simulink model "Automatic_Laser_Follower_Project"  (R2023b)
settings: Solver=ode45  StartTime=0.0  StopTime=100.0  RelTol=1e-3  EnableMultiTasking=on
undefined symbols (not defined in the file): fspecial, gray, none, Rec, SDTV, videoinput
libraries: visiontextngfix x11, visionconversions x4, visionanalysis x4, visionstatistics x3, simulink x3, imaqlib x1
settings Model: SimulationMode=accelerator  Creator=Chris  LastModifiedBy=fanyi
settings SolverCC: AlgebraicLoopSolver=TrustRegion
settings DataIOCC: LimitDataPoints=on  SaveFormat=Array  SignalLoggingSaveFormat=ModelDataLogs  ReturnWorkspaceOutputs=off
settings OptimizationCC: ExpressionDepthLimit=2147483647  LifeSpan=inf
settings DebuggingCC: UnderspecifiedInitializationDetection=Classic  MergeDetectMultiDrivingBlocksExec=none  SolverPrmCheckMsg=warning  FcnCallInpInsideContextMsg=warning  UnconnectedInputMsg=warning  UnconnectedOutputMsg=warning  UnconnectedLineMsg=warning  StateNameClashWarn=warning  SFUnexpectedBacktrackingDiag=warning  SFNoUnconditionalDefaultTransitionDiag=warning  SFExecutionAtInitializationDiag=none  ArithmeticOperatorsInVariantConditions=warning
settings HardwareCC: ProdBitPerPointer=32  ProdBitPerSizeT=32  ProdBitPerPtrDiffT=32  ProdLargestAtomicFloat=None  ProdIntDivRoundTo=Undefined  ProdEndianess=Unspecified  ProdWordSize=32  ProdHWDeviceType=32-bit Generic
settings ModelReferenceCC: EnableRefExpFcnMdlSchedulingChecks=on  PropagateSignalLabelsOutOfModel=off
settings SFSimCC: SimUseLocalCustomCode=off  CustomCodeUndefinedFunction=UseInterfaceOnly
settings RTWCC: RTWUseLocalCustomCode=off  DLArmComputeVersion=19.05
settings CodeAppCC: StateflowObjectComments=on
settings GRTTargetCC: TargetLangStandard=C89/C90 (ANSI)  CombineOutputUpdateFcns=off  GRTInterface=on
settings ConfigComp: CovMetricSettings=dw  CovSaveCumulativeToWorkspaceVar=on  CovSaveSingleToWorkspaceVar=on  CovExternalEMLEnable=off

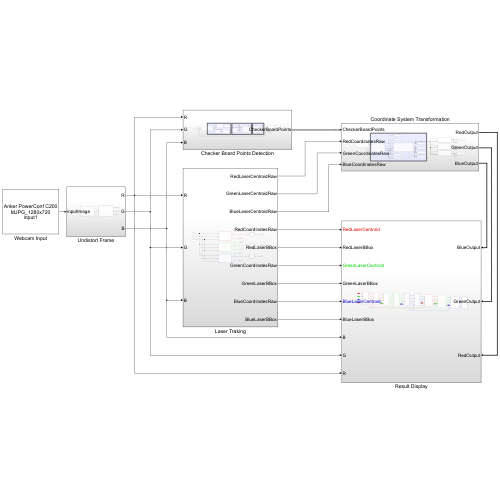
[thumbnail: Simulink's stored preview of the top-level diagram]
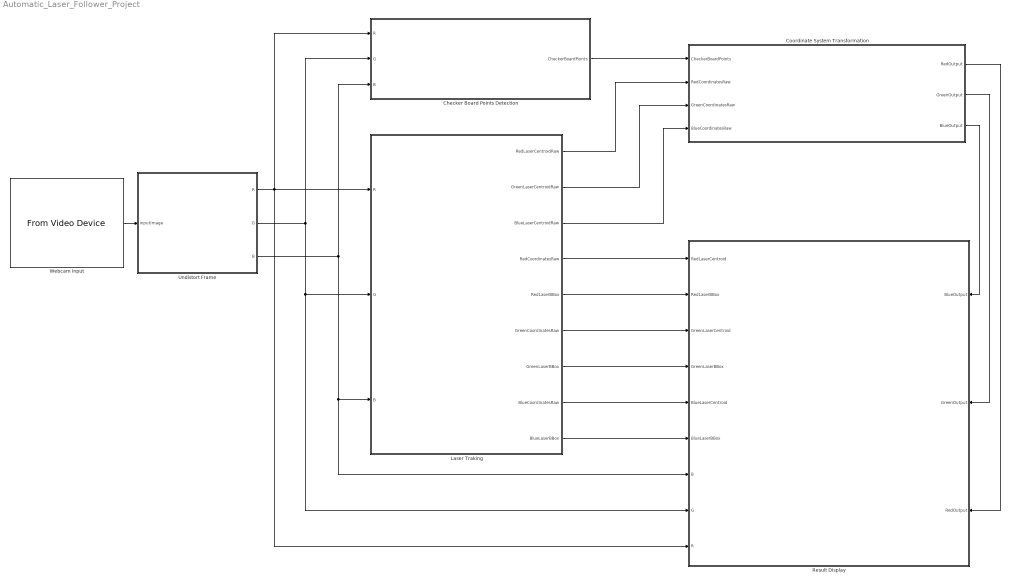
== system Automatic_Laser_Follower_Project ==
  Checker Board Points Detection : Subsystem
  Coordinate System Transformation : Subsystem
  Laser Traking : Subsystem
  Result Display : Subsystem
      settings: PortSchema="{\"entries\":[{\"content\":{\"sides\":[{\"content\":{\"connectorIds\":[\"In1\",\"In2\",\"In3\",\"In4\",\"In5\",\"In6\",\"In7\",\"In8\",\"In9\"]},\"type\":\"ConnectorPlacement.EquallySpacedRectSide\",\"uuid\":\"b1906bfe-0566-47b0-9e68-516326f7bec6\"},{\"content\":{\"connectorIds\":[\"In10\",\"In11\",\"In12\"],\"side\":\"RIGHT\"},\"type\":\"ConnectorPlacement.EquallySpacedRectSide\",\"uuid\":\"6258ed97-87fe-4cc0-87ce-9e8e3abb5e56\"},{\"content\":{\"side\":\"TOP\"},\"type\":\"ConnectorPlacement.EquallySpacedRectSide\",\"uuid\":\"7eb9bd65-632c-4cad-bc7f-e4ae4268f70b\"}]},\"type\":\"ConnectorPlacement.EquallySpacedConnector\",\"uuid\":\"5d2784b2-c65f-4f4f-828d-caa1666124b0\"}],\"packageUris\":[\"http://schema.mathworks.com/mf0/Connector/R2020b\"],\"version\":\"1.0\"}"
  Undistort Frame : Subsystem
  Webcam Input : imaqlib/From Video Device  DeviceMenu=winvideo 1 (Anker PowerConf C200)  Device=winvideo 1 (Anker PowerConf C200)  ObjConstructor=videoinput('winvideo', 1)  VideoFormatMenu=MJPG_1280x720  VideoFormat=MJPG_1280x720  VideoSource=input1  ROIPosition=[0 0 720 1280]  EnableHWTrigger=off  TriggerConfiguration=none/none  SampleTime=1/30  OutputPortsMode=One multidimensional signal  DataType=single  CanDoHWTrigger=no  ReturnedColorSpace=rgb  BlockHandle=1881.0001  ROIWidth=1280  ROIHeight=720  ROIColumn=0  ROIRow=0  EngXMLPath=C:\Program Files\MATLAB\R2023b\toolbox\imaq\imaq\private  DevXMLPath=C:\ProgramData\MATLAB\SupportPackages\R2023b\toolbox\imaq\supportpackages\genericvideo\adaptor\win64  EngLibPath=C:\Program Files\MATLAB\R2023b\toolbox\imaq\imaqblks\imaqmex\win64  ColorSpace=rgb  BayerSensorAlignment=grbg  ImaqMode=off
  wires:
  Checker Board Points Detection/1(CheckerBoardPoints) -> Coordinate System Transformation/1(CheckerBoardPoints)
  Coordinate System Transformation/1(RedOutput) -> Result Display/12(RedOutput)
  Coordinate System Transformation/3(BlueOutput) -> Result Display/10(BlueOutput)
  Coordinate System Transformation/2(GreenOutput) -> Result Display/11(GreenOutput)
  Laser Traking/4(RedCoordinatesRaw) -> Result Display/1(RedLaserCentroid)
  Laser Traking/5(RedLaserBBox) -> Result Display/2(RedLaserBBox)
  Laser Traking/6(GreenCoordinatesRaw) -> Result Display/3(GreenLaserCentroid)
  Laser Traking/7(GreenLaserBBox) -> Result Display/4(GreenLaserBBox)
  Laser Traking/8(BlueCoordinatesRaw) -> Result Display/5(BlueLaserCentroid)
  Laser Traking/9(BlueLaserBBox) -> Result Display/6(BlueLaserBBox)
  Laser Traking/1(RedLaserCentroidRaw) -> Coordinate System Transformation/2(RedCoordinatesRaw)
  Laser Traking/2(GreenLaserCentroidRaw) -> Coordinate System Transformation/3(GreenCoordinatesRaw)
  Laser Traking/3(BlueLaserCentroidRaw) -> Coordinate System Transformation/4(BlueCoordinatesRaw)
  Webcam Input/1 -> Undistort Frame/1(inputImage)
  Undistort Frame/2(G) -> Checker Board Points Detection/2(G), Result Display/8(G), Laser Traking/2(G)
  Undistort Frame/1(R) -> Checker Board Points Detection/1(R), Result Display/9(R), Laser Traking/1(R)
  Undistort Frame/3(B) -> Checker Board Points Detection/3(B), Result Display/7(B), Laser Traking/3(B)

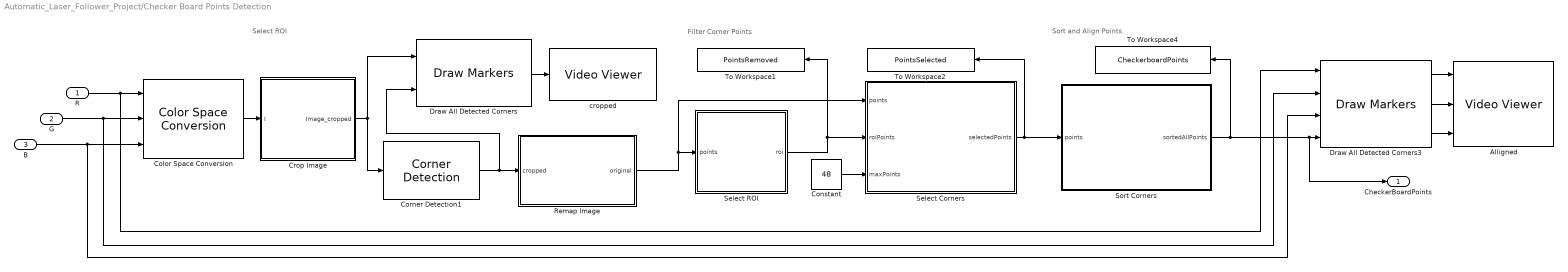
== system Automatic_Laser_Follower_Project/Checker Board Points Detection ==
  note: Sort and Align Points
  note: Select ROI
  note: Filter Corner Points
  R : Inport
  G : Inport  Port=2
  B : Inport  Port=3
  Alligned : VideoViewer  imagePorts=separate color signals  colormapValue=gray(256)  FigPos=[629.666666666667 1316.66666666667 1589.33333333333 1111.33333333333]
  Color Space Conversion : visionconversions/Color Space  Conversion  conversion=Obsolete  conversionActive=R'G'B' to intensity  wp_str=D65  rec=Rec. 601 (SDTV)  sys=1125/60/2:1  imagePorts=Separate color signals
  Constant : Constant  Value=48
  Corner Detection1 : visionanalysis/Corner Detection  method=Harris corner detection (Harris & Stephens)  factor=0.1  filter=fspecial('gaussian', [1 5], 1.5)  thrInten=0.1  thrAngle=157.5  output=Obsolete9b  outputInUse=Corner location  maxNum=80  thrMetric=0.0004  neighborSize=[21 21]  isOutVarDim=on  roundingMode=Floor  overflowMode=off  firstCoeffMode=Specify word length  firstCoeffWordLength=16  firstCoeffFracLength=16  prodOutputMode=Binary point scaling  prodOutputWordLength=32  prodOutputFracLength=0  accumMode=Binary point scaling  accumWordLength=32  accumFracLength=0  memoryMode=Binary point scaling  memoryWordLength=32  memoryFracLength=0
  Crop Image : MATLAB Function  TreatAsAtomicUnit=on
  Draw All Detected Corners : visiontextngfix/Draw Markers  shape=Circle  size=2  fill=on  fillClrSource=Specify via dialog  display=User-specified value  intensity=200  color=[250 0 0]  opacity=0.6  viewport=Entire image  antialiasing=off  inType=Obsolete  imagePorts=One multidimensional signal  roundingMode=Floor  overflowMode=off  memoryMode=Specify word length  memoryWordLength=16  memoryFracLength=15  prodOutputMode=Binary point scaling  prodOutputWordLength=32  prodOutputFracLength=14
  Draw All Detected Corners3 : visiontextngfix/Draw Markers  shape=Circle  size=2  fill=on  fillClrSource=Specify via dialog  display=User-specified value  intensity=200  color=[250 0 0]  opacity=0.6  viewport=Entire image  antialiasing=off  inType=Obsolete  imagePorts=Separate color signals  roundingMode=Floor  overflowMode=off  memoryMode=Specify word length  memoryWordLength=16  memoryFracLength=15  prodOutputMode=Binary point scaling  prodOutputWordLength=32  prodOutputFracLength=14
  Remap Image : MATLAB Function  TreatAsAtomicUnit=on
  Select Corners : MATLAB Function  TreatAsAtomicUnit=on
  Select ROI : MATLAB Function  TreatAsAtomicUnit=on
  Sort Corners : MATLAB Function  TreatAsAtomicUnit=on
  To Workspace1 : ToWorkspace  VariableName=PointsRemoved  SaveFormat=Structure With Time  SampleTime=-1
      settings: Save2DSignal=2-D array (concatenate along first dimension)
  To Workspace2 : ToWorkspace  VariableName=PointsSelected  SaveFormat=Structure With Time  SampleTime=-1
      settings: Save2DSignal=2-D array (concatenate along first dimension)
  To Workspace4 : ToWorkspace  VariableName=CheckerboardPoints  SaveFormat=Structure With Time  SampleTime=-1
      settings: Save2DSignal=2-D array (concatenate along first dimension)
  cropped : VideoViewer  colormapValue=gray(256)  FigPos=[1282.33333333333 1388.66666666667 1277.33333333333 1286]
  CheckerBoardPoints : Outport
  wires:
  G/1 -> Color Space Conversion/2, Draw All Detected Corners3/2
  B/1 -> Color Space Conversion/3, Draw All Detected Corners3/3
  R/1 -> Color Space Conversion/1, Draw All Detected Corners3/1
  Select ROI/1(roi) -> To Workspace1/1, Select Corners/2(roiPoints)
  Constant/1 -> Select Corners/3(maxPoints)
  Draw All Detected Corners3/2 -> Alligned/2
  Draw All Detected Corners3/3 -> Alligned/3
  Draw All Detected Corners3/1 -> Alligned/1
  Select Corners/1(selectedPoints) -> To Workspace2/1, Sort Corners/1(points)
  Draw All Detected Corners/1 -> cropped/1
  Color Space Conversion/1 -> Crop Image/1(I)
  Remap Image/1(original) -> Select Corners/1(points), Select ROI/1(points)
  Crop Image/1(Image_cropped) -> Corner Detection1/1, Draw All Detected Corners/1
  Corner Detection1/1 -> Remap Image/1(cropped), Draw All Detected Corners/2
  Sort Corners/1(sortedAllPoints) -> To Workspace4/1, Draw All Detected Corners3/4, CheckerBoardPoints/1

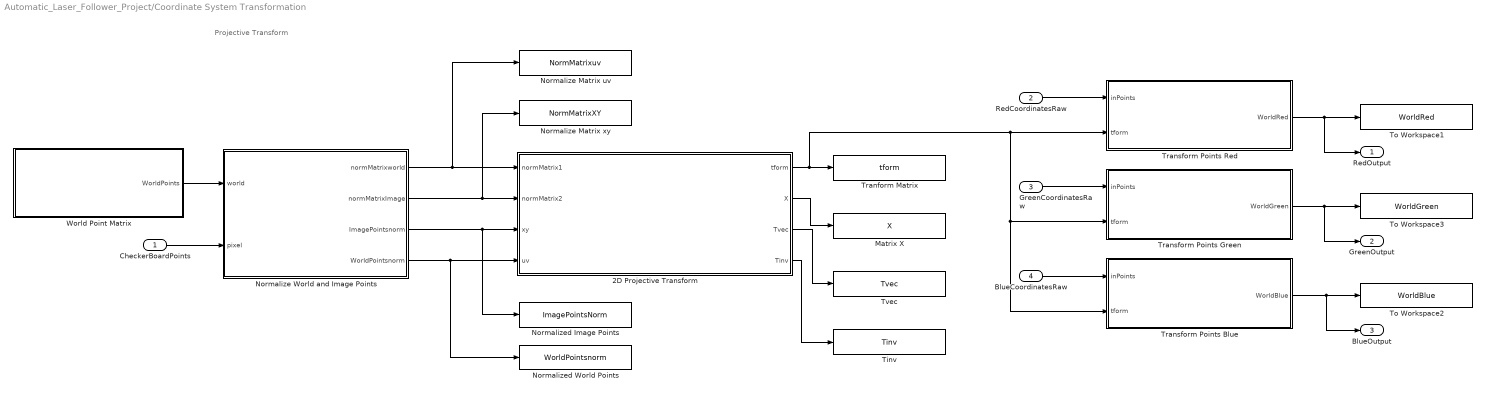
== system Automatic_Laser_Follower_Project/Coordinate System Transformation ==
  note: Projective Transform
  CheckerBoardPoints : Inport
  RedCoordinatesRaw : Inport  Port=2
  GreenCoordinatesRaw : Inport  Port=3
  BlueCoordinatesRaw : Inport  Port=4
  2D Projective Transform : MATLAB Function  TreatAsAtomicUnit=on
  Matrix X : ToWorkspace  VariableName=X  SaveFormat=Structure With Time  SampleTime=-1
      settings: Save2DSignal=2-D array (concatenate along first dimension)
  Normalize Matrix uv : ToWorkspace  VariableName=NormMatrixuv  SaveFormat=Structure With Time  SampleTime=-1
      settings: Save2DSignal=2-D array (concatenate along first dimension)
  Normalize Matrix xy : ToWorkspace  VariableName=NormMatrixXY  SaveFormat=Structure With Time  SampleTime=-1
      settings: Save2DSignal=2-D array (concatenate along first dimension)
  Normalize World and Image Points : MATLAB Function  TreatAsAtomicUnit=on
  Normalized Image Points : ToWorkspace  VariableName=ImagePointsNorm  SaveFormat=Structure With Time  SampleTime=-1
      settings: Save2DSignal=2-D array (concatenate along first dimension)
  Normalized World Points : ToWorkspace  VariableName=WorldPointsnorm  SaveFormat=Structure With Time  SampleTime=-1
      settings: Save2DSignal=2-D array (concatenate along first dimension)
  Tinv : ToWorkspace  VariableName=Tinv  SaveFormat=Structure With Time  SampleTime=-1
      settings: Save2DSignal=2-D array (concatenate along first dimension)
  To Workspace1 : ToWorkspace  VariableName=WorldRed  SaveFormat=Structure With Time  SampleTime=-1
      settings: Save2DSignal=2-D array (concatenate along first dimension)
  To Workspace2 : ToWorkspace  VariableName=WorldBlue  SaveFormat=Structure With Time  SampleTime=-1
      settings: Save2DSignal=2-D array (concatenate along first dimension)
  To Workspace3 : ToWorkspace  VariableName=WorldGreen  SaveFormat=Structure With Time  SampleTime=-1
      settings: Save2DSignal=2-D array (concatenate along first dimension)
  Tranform Matrix : ToWorkspace  VariableName=tform  SaveFormat=Structure With Time  SampleTime=-1
      settings: Save2DSignal=2-D array (concatenate along first dimension)
  Transform Points Blue : MATLAB Function  TreatAsAtomicUnit=on
  Transform Points Green : MATLAB Function  TreatAsAtomicUnit=on
  Transform Points Red : MATLAB Function  TreatAsAtomicUnit=on
  Tvec : ToWorkspace  VariableName=Tvec  SaveFormat=Structure With Time  SampleTime=-1
      settings: Save2DSignal=2-D array (concatenate along first dimension)
  World Point Matrix : MATLAB Function  TreatAsAtomicUnit=on
  RedOutput : Outport
  GreenOutput : Outport  Port=2
  BlueOutput : Outport  Port=3
  wires:
  Transform Points Red/1(WorldRed) -> RedOutput/1, To Workspace1/1
  Transform Points Green/1(WorldGreen) -> GreenOutput/1, To Workspace3/1
  Transform Points Blue/1(WorldBlue) -> To Workspace2/1, BlueOutput/1
  RedCoordinatesRaw/1 -> Transform Points Red/1(inPoints)
  GreenCoordinatesRaw/1 -> Transform Points Green/1(inPoints)
  BlueCoordinatesRaw/1 -> Transform Points Blue/1(inPoints)
  2D Projective Transform/1(tform) -> Tranform Matrix/1, Transform Points Blue/2(tform), Transform Points Green/2(tform), Transform Points Red/2(tform)
  CheckerBoardPoints/1 -> Normalize World and Image Points/2(pixel)
  Normalize World and Image Points/4(WorldPointsnorm) -> 2D Projective Transform/4(uv), Normalized World Points/1
  Normalize World and Image Points/2(normMatrixImage) -> Normalize Matrix xy/1, 2D Projective Transform/2(normMatrix2)
  Normalize World and Image Points/1(normMatrixworld) -> Normalize Matrix uv/1, 2D Projective Transform/1(normMatrix1)
  World Point Matrix/1(WorldPoints) -> Normalize World and Image Points/1(world)
  Normalize World and Image Points/3(ImagePointsnorm) -> Normalized Image Points/1, 2D Projective Transform/3(xy)
  2D Projective Transform/2(X) -> Matrix X/1
  2D Projective Transform/3(Tvec) -> Tvec/1
  2D Projective Transform/4(Tinv) -> Tinv/1

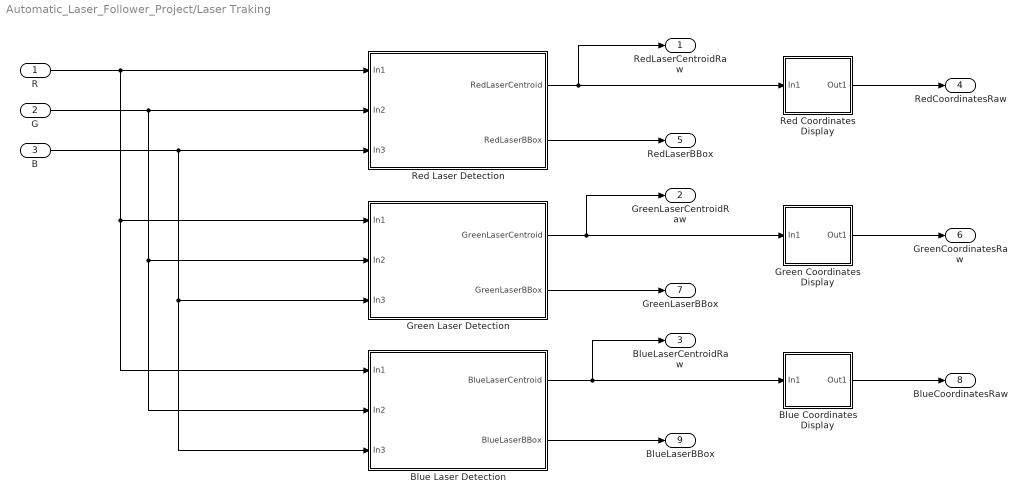
== system Automatic_Laser_Follower_Project/Laser Traking ==
  R : Inport
  G : Inport  Port=2
  B : Inport  Port=3
  Blue Coordinates Display : Subsystem
  Blue Laser Detection : Subsystem
  Green Coordinates Display : Subsystem
  Green Laser Detection : Subsystem
  Red Coordinates Display : Subsystem
  Red Laser Detection : Subsystem  VariantControl=Choice
  RedLaserCentroidRaw : Outport
  GreenLaserCentroidRaw : Outport  Port=2
  BlueLaserCentroidRaw : Outport  Port=3
  RedCoordinatesRaw : Outport  Port=4
  RedLaserBBox : Outport  Port=5
  GreenCoordinatesRaw : Outport  Port=6
  GreenLaserBBox : Outport  Port=7
  BlueCoordinatesRaw : Outport  Port=8
  BlueLaserBBox : Outport  Port=9
  wires:
  Blue Laser Detection/2(BlueLaserBBox) -> BlueLaserBBox/1
  Green Laser Detection/1(GreenLaserCentroid) -> Green Coordinates Display/1(In1), GreenLaserCentroidRaw/1
  Red Laser Detection/1(RedLaserCentroid) -> Red Coordinates Display/1(In1), RedLaserCentroidRaw/1
  Blue Laser Detection/1(BlueLaserCentroid) -> BlueLaserCentroidRaw/1, Blue Coordinates Display/1(In1)
  Red Laser Detection/2(RedLaserBBox) -> RedLaserBBox/1
  Red Coordinates Display/1(Out1) -> RedCoordinatesRaw/1
  Green Coordinates Display/1(Out1) -> GreenCoordinatesRaw/1
  Blue Coordinates Display/1(Out1) -> BlueCoordinatesRaw/1
  G/1 -> Green Laser Detection/2(In2), Blue Laser Detection/2(In2), Red Laser Detection/2(In2)
  Green Laser Detection/2(GreenLaserBBox) -> GreenLaserBBox/1
  R/1 -> Blue Laser Detection/1(In1), Green Laser Detection/1(In1), Red Laser Detection/1(In1)
  B/1 -> Blue Laser Detection/3(In3), Green Laser Detection/3(In3), Red Laser Detection/3(In3)

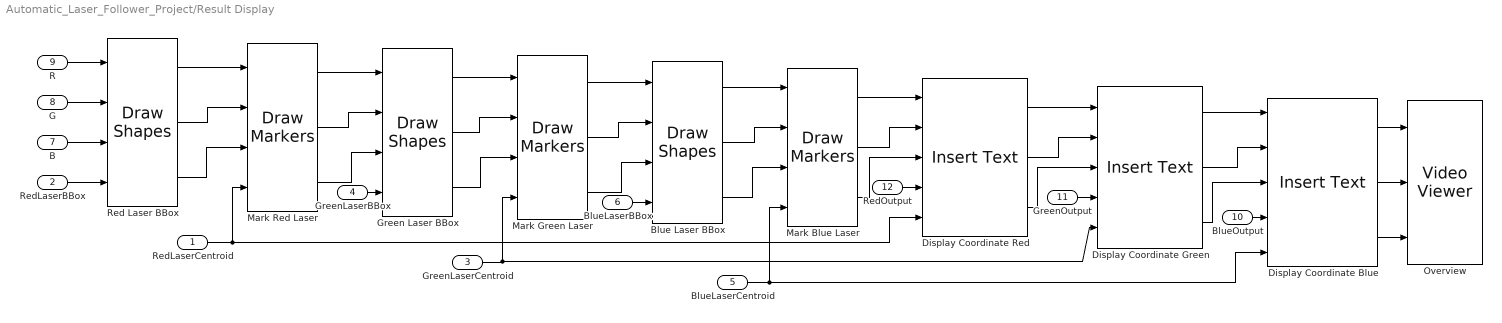
== system Automatic_Laser_Follower_Project/Result Display ==
  RedLaserCentroid : Inport
  RedLaserBBox : Inport  Port=2
  GreenLaserCentroid : Inport  Port=3
  GreenLaserBBox : Inport  Port=4
  BlueLaserCentroid : Inport  Port=5
  BlueLaserBBox : Inport  Port=6
  B : Inport  Port=7
  G : Inport  Port=8
  R : Inport  Port=9
  BlueOutput : Inport  Port=10
  GreenOutput : Inport  Port=11
  RedOutput : Inport  Port=12
  Blue Laser BBox : visiontextngfix/Draw Shapes  shape=Rectangles  fill=off  lineWidth=3  fillClrSource=Specify via dialog  display=User-specified value  intensity=200  color=[0 0 255]  opacity=0.6  viewport=Entire image  antialiasing=off  inType=Obsolete  imagePorts=Separate color signals  roundingMode=Floor  overflowMode=off  memoryMode=Specify word length  memoryWordLength=16  prodOutputMode=Binary point scaling  prodOutputWordLength=32  prodOutputFracLength=14  memoryFracLength=15
  Display Coordinate Blue : visiontextngfix/Insert Text  inputType=Obsolete  theText='blue: %.3f mm, %.3f mm'  getTextLocFrom=Input port  textLoc=[1 1]  getTextColorFrom=Specify via dialog  textColor=[0 0 255]  getTextIntensityFrom=Specify via dialog  textIntensity=0  getTextOpacityFrom=Specify via dialog  textOpacity=1.0  dummyVar2=0  dummyVar3=0  dummyVar4=0  imagePorts=Separate color signals  isInputTransposed=off  fontFace=LucidaSansRegular  dummyVar1=0  blockFontSize=18  antiAliased=on
  Display Coordinate Green : visiontextngfix/Insert Text  inputType=Obsolete  theText='Green: %.3f mm, %.3f mm'  getTextLocFrom=Input port  textLoc=[1 1]  getTextColorFrom=Specify via dialog  textColor=[0 255 0]  getTextIntensityFrom=Specify via dialog  textIntensity=0  getTextOpacityFrom=Specify via dialog  textOpacity=1.0  dummyVar2=0  dummyVar3=0  dummyVar4=0  imagePorts=Separate color signals  isInputTransposed=off  fontFace=LucidaSansRegular  dummyVar1=0  blockFontSize=18  antiAliased=on
  Display Coordinate Red : visiontextngfix/Insert Text  inputType=Obsolete  theText='Red: %.3f mm, %.3f mm'  getTextLocFrom=Input port  textLoc=[1 1]  getTextColorFrom=Specify via dialog  textColor=[255 0 0]  getTextIntensityFrom=Specify via dialog  textIntensity=0  getTextOpacityFrom=Specify via dialog  textOpacity=1.0  dummyVar2=0  dummyVar3=0  dummyVar4=0  imagePorts=Separate color signals  isInputTransposed=off  fontFace=LucidaSansRegular  dummyVar1=0  blockFontSize=18  antiAliased=on
  Green Laser BBox : visiontextngfix/Draw Shapes  shape=Rectangles  fill=off  lineWidth=3  fillClrSource=Specify via dialog  display=User-specified value  intensity=200  color=[0 255 0]  opacity=0.6  viewport=Entire image  antialiasing=off  inType=Obsolete  imagePorts=Separate color signals  roundingMode=Floor  overflowMode=off  memoryMode=Specify word length  memoryWordLength=16  prodOutputMode=Binary point scaling  prodOutputWordLength=32  prodOutputFracLength=14  memoryFracLength=15
  Mark Blue Laser : visiontextngfix/Draw Markers  shape=X-mark  size=5  fill=on  fillClrSource=Specify via dialog  display=User-specified value  intensity=200  color=[0 0 255]  opacity=0.6  viewport=Entire image  antialiasing=off  inType=Obsolete  imagePorts=Separate color signals  roundingMode=Floor  overflowMode=off  memoryMode=Specify word length  memoryWordLength=16  memoryFracLength=15  prodOutputMode=Binary point scaling  prodOutputWordLength=32  prodOutputFracLength=14
  Mark Green Laser : visiontextngfix/Draw Markers  shape=X-mark  size=5  fill=on  fillClrSource=Specify via dialog  display=User-specified value  intensity=200  color=[0 255 0]  opacity=0.6  viewport=Entire image  antialiasing=off  inType=Obsolete  imagePorts=Separate color signals  roundingMode=Floor  overflowMode=off  memoryMode=Specify word length  memoryWordLength=16  memoryFracLength=15  prodOutputMode=Binary point scaling  prodOutputWordLength=32  prodOutputFracLength=14
  Mark Red Laser : visiontextngfix/Draw Markers  shape=X-mark  size=5  fill=on  fillClrSource=Specify via dialog  display=User-specified value  intensity=200  color=[255 0 0]  opacity=0.6  viewport=Entire image  antialiasing=off  inType=Obsolete  imagePorts=Separate color signals  roundingMode=Floor  overflowMode=off  memoryMode=Specify word length  memoryWordLength=16  memoryFracLength=15  prodOutputMode=Binary point scaling  prodOutputWordLength=32  prodOutputFracLength=14
  Overview : VideoViewer  imagePorts=separate color signals  colormapValue=gray(256)  FigPos=[1 1390 2560 1294.66666666667]
  Red Laser BBox : visiontextngfix/Draw Shapes  shape=Rectangles  fill=off  lineWidth=3  fillClrSource=Specify via dialog  display=User-specified value  intensity=200  color=[255 0 0]  opacity=0.6  viewport=Entire image  antialiasing=off  inType=Obsolete  imagePorts=Separate color signals  roundingMode=Floor  overflowMode=off  memoryMode=Specify word length  memoryWordLength=16  prodOutputMode=Binary point scaling  prodOutputWordLength=32  prodOutputFracLength=14  memoryFracLength=15
  wires:
  RedLaserBBox/1 -> Red Laser BBox/4
  Mark Green Laser/1 -> Blue Laser BBox/1
  Green Laser BBox/3 -> Mark Green Laser/3
  Mark Green Laser/2 -> Blue Laser BBox/2
  Mark Green Laser/3 -> Blue Laser BBox/3
  Display Coordinate Green/3 -> Display Coordinate Blue/3
  Mark Blue Laser/1 -> Display Coordinate Red/1
  Green Laser BBox/1 -> Mark Green Laser/1
  Display Coordinate Green/2 -> Display Coordinate Blue/2
  Display Coordinate Red/1 -> Display Coordinate Green/1
  Blue Laser BBox/1 -> Mark Blue Laser/1
  Display Coordinate Green/1 -> Display Coordinate Blue/1
  Blue Laser BBox/3 -> Mark Blue Laser/3
  Red Laser BBox/3 -> Mark Red Laser/3
  Red Laser BBox/2 -> Mark Red Laser/2
  Mark Red Laser/3 -> Green Laser BBox/3
  Mark Blue Laser/2 -> Display Coordinate Red/2
  Mark Red Laser/2 -> Green Laser BBox/2
  Green Laser BBox/2 -> Mark Green Laser/2
  Red Laser BBox/1 -> Mark Red Laser/1
  Display Coordinate Red/3 -> Display Coordinate Green/3
  RedLaserCentroid/1 -> Mark Red Laser/4, Display Coordinate Red/5
  Blue Laser BBox/2 -> Mark Blue Laser/2
  Display Coordinate Red/2 -> Display Coordinate Green/2
  R/1 -> Red Laser BBox/1
  Mark Blue Laser/3 -> Display Coordinate Red/3
  BlueLaserBBox/1 -> Blue Laser BBox/4
  B/1 -> Red Laser BBox/3
  GreenLaserBBox/1 -> Green Laser BBox/4
  Mark Red Laser/1 -> Green Laser BBox/1
  GreenLaserCentroid/1 -> Display Coordinate Green/5, Mark Green Laser/4
  BlueLaserCentroid/1 -> Mark Blue Laser/4, Display Coordinate Blue/5
  G/1 -> Red Laser BBox/2
  Display Coordinate Blue/1 -> Overview/1
  Display Coordinate Blue/2 -> Overview/2
  Display Coordinate Blue/3 -> Overview/3
  RedOutput/1 -> Display Coordinate Red/4
  BlueOutput/1 -> Display Coordinate Blue/4
  GreenOutput/1 -> Display Coordinate Green/4

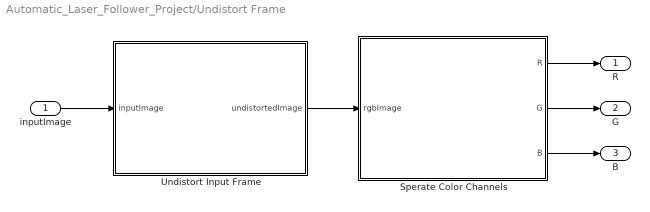
== system Automatic_Laser_Follower_Project/Undistort Frame ==
  inputImage : Inport
  Sperate Color Channels : MATLAB Function  TreatAsAtomicUnit=on
  Undistort Input Frame : MATLAB Function  TreatAsAtomicUnit=on
  R : Outport
  G : Outport  Port=2
  B : Outport  Port=3
  wires:
  Sperate Color Channels/2(G) -> G/1
  Sperate Color Channels/3(B) -> B/1
  Sperate Color Channels/1(R) -> R/1
  inputImage/1 -> Undistort Input Frame/1(inputImage)
  Undistort Input Frame/1(undistortedImage) -> Sperate Color Channels/1(rgbImage)

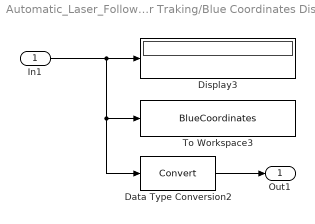
== system Automatic_Laser_Follower_Project/Laser Traking/Blue Coordinates Display ==
  In1 : Inport
  Data Type Conversion2 : DataTypeConversion  ConvertRealWorld=Stored Integer (SI)  SaturateOnIntegerOverflow=off  RndMeth=Floor
  Display3 : Display
  To Workspace3 : ToWorkspace  VariableName=BlueCoordinates  SampleTime=-1
      settings: Save2DSignal=2-D array (concatenate along first dimension)
  Out1 : Outport
  wires:
  In1/1 -> Data Type Conversion2/1, To Workspace3/1, Display3/1
  Data Type Conversion2/1 -> Out1/1

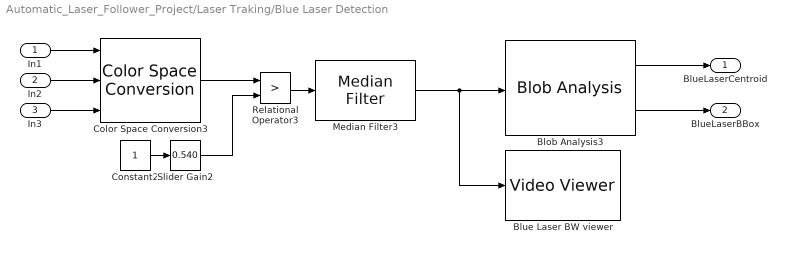
== system Automatic_Laser_Follower_Project/Laser Traking/Blue Laser Detection ==
  In1 : Inport
  In2 : Inport  Port=2
  In3 : Inport  Port=3
  Blob Analysis3 : visionstatistics/Blob Analysis  Tag=vipblks_row_conv  area=off  centroid=on  bBox=on  majorAxis=off  minorAxis=off  angle=off  eccentricity=off  equivDiameterSq=off  extent=off  perimeter=off  outDT=double  conn=8  isLabel=off  maxBlobs=1  warnIfNumBlobsExceeded=on  isCount=off  useMinArea=on  minArea=40  useMaxArea=on  maxArea=intmax('uint32')  excludeBorderBlob=off  isOutVarDim=off  isFill=on  fillValues=-1  roundingMode=Floor  overflowMode=off  prodOutputMode=Binary point scaling  prodOutputWordLength=32  prodOutputFracLength=16  accumMode=Binary point scaling  accumWordLength=32  accumFracLength=0  outputMode=Binary point scaling  outputWordLength=32  outputFracLength=16  firstCoeffMode=Binary point scaling  firstCoeffWordLength=16  firstCoeffFracLength=14  secondCoeffMode=Binary point scaling  secondCoeffWordLength=32  secondCoeffFracLength=16
  Blue Laser BW viewer : VideoViewer  colormapValue=gray(256)  FigPos=[933 1177.33333333333 1538 856.666666666667]
  Color Space Conversion3 : visionconversions/Color Space  Conversion  conversion=Obsolete  conversionActive=R'G'B' to Y'CbCr  wp_str=D65  rec=Rec. 601 (SDTV)  sys=1125/60/2:1  imagePorts=Separate color signals
  Constant2 : Constant
  Median Filter3 : visionanalysis/Median Filter  nghbood=ones(1, 1)  outSize=Valid  padType=Constant  padSrc=Specify via dialog  padVal=0  roundingMode=Floor  overflowMode=off
  Relational Operator3 : RelationalOperator  Operator=>  OutDataTypeStr=boolean  RndMeth=Simplest  InputSameDT=off
  Slider Gain2 : simulink/Math Operations/Slider Gain  gain=0.540  low=0  high=1
  BlueLaserCentroid : Outport
  BlueLaserBBox : Outport  Port=2
  wires:
  Slider Gain2/1 -> Relational Operator3/2
  Median Filter3/1 -> Blob Analysis3/1, Blue Laser BW viewer/1
  In2/1 -> Color Space Conversion3/2
  Constant2/1 -> Slider Gain2/1
  Relational Operator3/1 -> Median Filter3/1
  Color Space Conversion3/2 -> Relational Operator3/1
  Blob Analysis3/1 -> BlueLaserCentroid/1
  In1/1 -> Color Space Conversion3/1
  Blob Analysis3/2 -> BlueLaserBBox/1
  In3/1 -> Color Space Conversion3/3

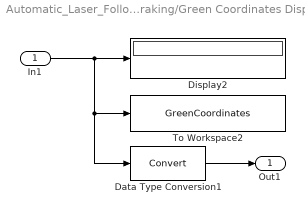
== system Automatic_Laser_Follower_Project/Laser Traking/Green Coordinates Display ==
  In1 : Inport
  Data Type Conversion1 : DataTypeConversion  ConvertRealWorld=Stored Integer (SI)  SaturateOnIntegerOverflow=off  RndMeth=Floor
  Display2 : Display
  To Workspace2 : ToWorkspace  VariableName=GreenCoordinates  SampleTime=-1
      settings: Save2DSignal=2-D array (concatenate along first dimension)
  Out1 : Outport
  wires:
  Data Type Conversion1/1 -> Out1/1
  In1/1 -> Data Type Conversion1/1, To Workspace2/1, Display2/1

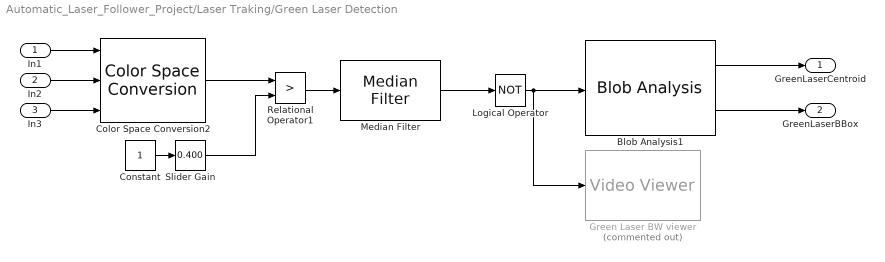
== system Automatic_Laser_Follower_Project/Laser Traking/Green Laser Detection ==
  In1 : Inport
  In2 : Inport  Port=2
  In3 : Inport  Port=3
  Blob Analysis1 : visionstatistics/Blob Analysis  Tag=vipblks_row_conv  area=off  centroid=on  bBox=on  majorAxis=off  minorAxis=off  angle=off  eccentricity=off  equivDiameterSq=off  extent=off  perimeter=off  outDT=double  conn=8  isLabel=off  maxBlobs=1  warnIfNumBlobsExceeded=on  isCount=off  useMinArea=on  minArea=0  useMaxArea=on  maxArea=intmax('uint32')  excludeBorderBlob=off  isOutVarDim=off  isFill=on  fillValues=-1  roundingMode=Floor  overflowMode=off  prodOutputMode=Binary point scaling  prodOutputWordLength=32  prodOutputFracLength=16  accumMode=Binary point scaling  accumWordLength=32  accumFracLength=0  outputMode=Binary point scaling  outputWordLength=32  outputFracLength=16  firstCoeffMode=Binary point scaling  firstCoeffWordLength=16  firstCoeffFracLength=14  secondCoeffMode=Binary point scaling  secondCoeffWordLength=32  secondCoeffFracLength=16
  Color Space Conversion2 : visionconversions/Color Space  Conversion  conversion=Obsolete  conversionActive=R'G'B' to Y'CbCr  wp_str=D65  rec=Rec. 601 (SDTV)  sys=1125/60/2:1  imagePorts=Separate color signals
  Constant : Constant
  Green Laser BW viewer : VideoViewer  Commented=on  colormapValue=gray(256)  FigPos=[991.666666666667 959.333333333333 1476 664]
  Logical Operator : Logic  Operator=NOT  AllPortsSameDT=off  OutDataTypeStr=boolean
  Median Filter : visionanalysis/Median Filter  nghbood=ones(1, 1)  outSize=Valid  padType=Constant  padSrc=Specify via dialog  padVal=0  roundingMode=Floor  overflowMode=off
  Relational Operator1 : RelationalOperator  Operator=>  OutDataTypeStr=boolean  RndMeth=Simplest  InputSameDT=off
  Slider Gain : simulink/Math Operations/Slider Gain  gain=0.400  low=0  high=1
  GreenLaserCentroid : Outport
  GreenLaserBBox : Outport  Port=2
  wires:
  Blob Analysis1/2 -> GreenLaserBBox/1
  Relational Operator1/1 -> Median Filter/1
  Slider Gain/1 -> Relational Operator1/2
  Median Filter/1 -> Logical Operator/1
  Color Space Conversion2/2 -> Relational Operator1/1
  In3/1 -> Color Space Conversion2/3
  Constant/1 -> Slider Gain/1
  In2/1 -> Color Space Conversion2/2
  In1/1 -> Color Space Conversion2/1
  Blob Analysis1/1 -> GreenLaserCentroid/1
  Logical Operator/1 -> Green Laser BW viewer/1, Blob Analysis1/1

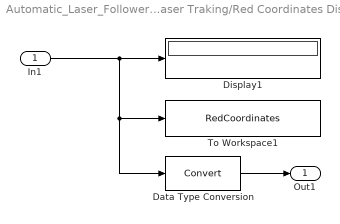
== system Automatic_Laser_Follower_Project/Laser Traking/Red Coordinates Display ==
  In1 : Inport
  Data Type Conversion : DataTypeConversion  ConvertRealWorld=Stored Integer (SI)  SaturateOnIntegerOverflow=off  RndMeth=Floor
  Display1 : Display
  To Workspace1 : ToWorkspace  VariableName=RedCoordinates  SampleTime=-1
      settings: Save2DSignal=2-D array (concatenate along first dimension)
  Out1 : Outport
  wires:
  In1/1 -> Data Type Conversion/1, To Workspace1/1, Display1/1
  Data Type Conversion/1 -> Out1/1

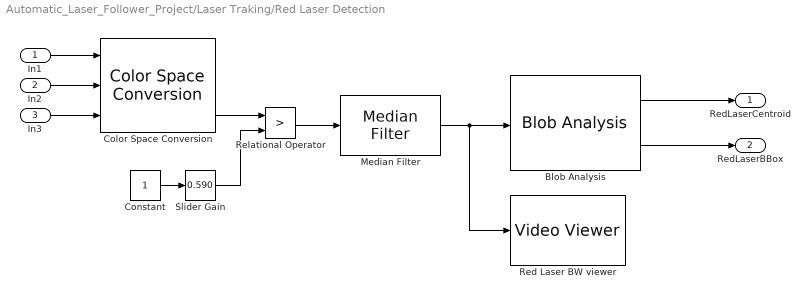
== system Automatic_Laser_Follower_Project/Laser Traking/Red Laser Detection ==
  In1 : Inport
  In2 : Inport  Port=2
  In3 : Inport  Port=3
  Blob Analysis : visionstatistics/Blob Analysis  Tag=vipblks_row_conv  area=off  centroid=on  bBox=on  majorAxis=off  minorAxis=off  angle=off  eccentricity=off  equivDiameterSq=off  extent=off  perimeter=off  outDT=double  conn=8  isLabel=off  maxBlobs=1  warnIfNumBlobsExceeded=on  isCount=off  useMinArea=on  minArea=0  useMaxArea=on  maxArea=intmax('uint32')  excludeBorderBlob=off  isOutVarDim=off  isFill=on  fillValues=-1  roundingMode=Floor  overflowMode=off  prodOutputMode=Binary point scaling  prodOutputWordLength=32  prodOutputFracLength=16  accumMode=Binary point scaling  accumWordLength=32  accumFracLength=0  outputMode=Binary point scaling  outputWordLength=32  outputFracLength=16  firstCoeffMode=Binary point scaling  firstCoeffWordLength=16  firstCoeffFracLength=14  secondCoeffMode=Binary point scaling  secondCoeffWordLength=32  secondCoeffFracLength=16
  Color Space Conversion : visionconversions/Color Space  Conversion  conversion=Obsolete  conversionActive=R'G'B' to Y'CbCr  wp_str=D65  rec=Rec. 601 (SDTV)  sys=1125/60/2:1  imagePorts=Separate color signals
  Constant : Constant
  Median Filter : visionanalysis/Median Filter  nghbood=ones(1, 1)  outSize=Valid  padType=Constant  padSrc=Specify via dialog  padVal=0  roundingMode=Floor  overflowMode=off
  Red Laser BW viewer : VideoViewer  colormapValue=gray(256)  FigPos=[9 1382 2544 1278.66666666667]
  Relational Operator : RelationalOperator  Operator=>  OutDataTypeStr=boolean  RndMeth=Simplest  InputSameDT=off
  Slider Gain : simulink/Math Operations/Slider Gain  gain=0.590  low=0  high=1
  RedLaserCentroid : Outport
  RedLaserBBox : Outport  Port=2
  wires:
  In2/1 -> Color Space Conversion/2
  In3/1 -> Color Space Conversion/3
  Median Filter/1 -> Blob Analysis/1, Red Laser BW viewer/1
  Relational Operator/1 -> Median Filter/1
  Constant/1 -> Slider Gain/1
  Slider Gain/1 -> Relational Operator/2
  Color Space Conversion/3 -> Relational Operator/1
  Blob Analysis/2 -> RedLaserBBox/1
  In1/1 -> Color Space Conversion/1
  Blob Analysis/1 -> RedLaserCentroid/1

== matlab function Automatic_Laser_Follower_Project/Coordinate System Transformation/Transform Points Red ==
  data: inPoints input; WorldRed output size=[1;2]; tform input
function WorldRed = TransformPointsInverseRed(inPoints, tform)

invtform = inv(tform);

homogPoints = [inPoints, ones(size(inPoints, 1), 1)];

transformedPoints = homogPoints * invtform'; 

% Normalize back to Cartesian coordinates
WorldRed = transformedPoints(:, 1:2) ./ transformedPoints(:, 3);


end

== matlab function Automatic_Laser_Follower_Project/Coordinate System Transformation/Transform Points Green ==
  data: inPoints input; WorldGreen output size=[1;2]; tform input
function WorldGreen = TransformPointsInverseGreen(inPoints, tform)

invtform = inv(tform);

homogPoints = [inPoints, ones(size(inPoints, 1), 1)];

transformedPoints = homogPoints * invtform'; 

% Normalize back to Cartesian coordinates
WorldGreen = transformedPoints(:, 1:2) ./ transformedPoints(:, 3);


end

== matlab function Automatic_Laser_Follower_Project/Checker Board Points Detection/Select Corners ==
  data: points input; roiPoints input size=[80;2]; selectedPoints output size=[80 2]; maxPoints input
function selectedPoints = selectCorners(points, roiPoints, maxPoints)
    %#codegen
    
    % Ensures the inputs are in the correct format
    assert(size(points, 2) == size(roiPoints, 2));
    
    % Using setdiff to find the points not in the ROI 
    selectedPoints = setdiff(points, roiPoints, 'rows', 'stable');
    
    % Makes sure the points selected does not overflow  
    if size(selectedPoints, 1) > maxPoints
        selectedPoints = selectedPoints(1:maxPoints, :);
    end
end

== matlab function Automatic_Laser_Follower_Project/Checker Board Points Detection/Select ROI ==
  data: points input size=[80;2]; roi output uint32 size=[80;2]
function roi = selectROI(points)
    %#codegen
    assert(size(points, 2) == 2, 'Input points must have exactly two columns'); % Assert input size
    
    points = double(points);
    
    % Calculates the convex hull of the points detected
    K = convhull(points(:,1), points(:,2));
    
    % Initialize a array for points touching or close to the convex hull
    isTouchingHull = false(size(points, 1), 1);
    
    % Define a threshold distance for points to be excluded in the ROI 
    threshold = 10; 

    % Loop over each segment of the convex hull
    for i = 1:numel(K)-1
        P1 = points(K(i), :);
        P2 = points(K(i+1), :);
        edgeVector = P2 - P1;

        for j = 1:size(points, 1)
            if ~isTouchingHull(j) % Only check points not already touching the hull
                pointVector = points(j, :) - P1;
                crossVec = norm(cross([pointVector 0], [edgeVector 0]));
                edgeLength = norm(edgeVector);
                distanceToEdge = crossVec / edgeLength;

                if distanceToEdge < threshold
                    isTouchingHull(j) = true;
                end
            end
        end
    end

    % Include points that are part of the hull or touching the hull
    isTouchingHull(K) = true;

    % Extract the points based on the logical index to be excluded in ROI 
    roiPoints = points(isTouchingHull, :);

    roi = uint32(roiPoints);
    
    assert(size(roi, 2) == 2);
end

== matlab function Automatic_Laser_Follower_Project/Checker Board Points Detection/Sort Corners ==
  data: points input; sortedAllPoints output size=[48;2]
function sortedAllPoints = sortCheckerboardPoints(points)
    points = double(points);

    % Remove rows with NaN values to clean the input data
    points = points(~any(isnan(points), 2), :);

    numRows = 6; 
    numCols = 8; 

    % Initialize the sorted points array
    sortedAllPoints = NaN(numRows * numCols, 2); 
    
    % Use kmeans to cluster points based on x-coordinate with PlusPlus initialization
    opts = statset('UseParallel', true, 'MaxIter', 1000);
    [idx, C] = kmeans(points(:,1), numCols, 'Options', opts, 'Distance', 'sqEuclidean', 'Replicates', 5, 'Start', 'plus');

    % Sort the centroids of clusters to ensure the order of clusters is from left to right
    [~, centroidOrder] = sort(C);
    
    % Initialize an index to keep track of where to insert points into sortedAllPoints
    insertIndex = 1;
    
    % Sort points within each cluster based on y-coordinate
    for i = 1:numCols
        % Find the points in the current cluster
        clusterPoints = points(idx == centroidOrder(i), :);
        
        % Sort the points in this cluster by their y-coordinate
        [~, order] = sort(clusterPoints(:,2), 'ascend');
        sortedClusterPoints = clusterPoints(order, :);
            
    % Dynamically handle missing or extra points in a cluster
    numPointsInCluster = size(sortedClusterPoints, 1);
    if numPointsInCluster >= numRows
        % If there are enough points, take the top numRows points
        sortedClusterPoints = sortedClusterPoints(1:numRows, :);
    else
        % If there are missing points, append NaN rows to make up the difference
        rowsToAdd = numRows - numPointsInCluster;
        if rowsToAdd > 0
            nanRows = NaN(rowsToAdd, 2);
            sortedClusterPoints = [sortedClusterPoints; nanRows];
        end
    end
        
        % Insert sorted points into the sortedAllPoints array
        sortedAllPoints(insertIndex:insertIndex + numRows - 1, :) = sortedClusterPoints;
        insertIndex = insertIndex + numRows;
    end
end

== matlab function Automatic_Laser_Follower_Project/Undistort Frame/Sperate Color Channels ==
  data: rgbImage input; R output; G output; B output
function [R, G, B] = separateColorChannels(rgbImage)
    % Check if the input image is indeed an RGB image
    if size(rgbImage, 3) ~= 3
        error('Input must be an RGB image.');
    end

    % Separate the color channels
    R = rgbImage(:, :, 1); 
    G = rgbImage(:, :, 2);  
    B = rgbImage(:, :, 3);  
end

== matlab function Automatic_Laser_Follower_Project/Checker Board Points Detection/Crop Image ==
  data: I input; Image_cropped output
function Image_cropped = cropImage(I)
    % cropping region
    rowStart = 300;
    rowEnd = 600;
    colStart = 300;
    colEnd = 600;

    Image_cropped = I(rowStart:rowEnd, colStart:colEnd);
end

== matlab function Automatic_Laser_Follower_Project/Checker Board Points Detection/Remap Image ==
  data: cropped input; original output size=[80;2]
function original = mapPointsToOriginal(cropped)
    rowOffset = 300 - 1;
    colOffset = 300 - 1;
    
    original = zeros(size(cropped));
    
    % Map each cropped point back to its original position
    for i = 1:size(cropped, 1)
        original(i, 1) = cropped(i, 1) + colOffset;
        original(i, 2) = cropped(i, 2) + rowOffset;
    end
end

== matlab function Automatic_Laser_Follower_Project/Undistort Frame/Undistort Input Frame ==
  data: inputImage input; undistortedImage output
function undistortedImage = undistortImage(inputImage)
    % Store the intrinsic matrix K
    intrinsicMatrix = [1025.30186847282, 0, 659.328530484529;
                       0, 1028.22633873043, 350.911761479516;
                       0, 0, 1];
    
    % Store the radial distortion coefficients
    k1 = 0.146451856840480;
    k2 = -0.129982636042747;
    
    % Initialize the undistorted image
    undistortedImage = zeros(size(inputImage), 'like', inputImage);
    
    % Get the number of rows and columns in the image
    [rows, cols, ~] = size(inputImage);
    
    for u = 1:cols
        for v = 1:rows
            % Convert pixel coordinates to normalized image coordinates
            x = (u - intrinsicMatrix(1,3)) / intrinsicMatrix(1,1);
            y = (v - intrinsicMatrix(2,3)) / intrinsicMatrix(2,2);
            
            % Compute the radius squared
            rSquared = x^2 + y^2;
            
            % Compute the undistortion factor
            undistortFactor = 1 + k1 * rSquared + k2 * rSquared^2;
            
            % Compute the undistorted coordinates
            xUndistorted = x * undistortFactor;
            yUndistorted = y * undistortFactor;
            
            % Convert back to pixel coordinates
            uUndistorted = round(xUndistorted * intrinsicMatrix(1,1) + intrinsicMatrix(1,3));
            vUndistorted = round(yUndistorted * intrinsicMatrix(2,2) + intrinsicMatrix(2,3));
            
            % Ensure the coordinates are within the image bounds
            if (uUndistorted > 0 && uUndistorted <= cols && vUndistorted > 0 && vUndistorted <= rows)
                undistortedImage(v, u, :) = inputImage(vUndistorted, uUndistorted, :);
            end
        end
    end
end

== matlab function Automatic_Laser_Follower_Project/Coordinate System Transformation/Transform Points Blue ==
  data: inPoints input; WorldBlue output size=[1;2]; tform input
function WorldBlue = TransformPointsInverseBlue(inPoints, tform)

invtform = inv(tform);

homogPoints = [inPoints, ones(size(inPoints, 1), 1)];

transformedPoints = homogPoints * invtform'; 

% Normalize back to Cartesian coordinates
WorldBlue = transformedPoints(:, 1:2) ./ transformedPoints(:, 3);


end

== matlab function Automatic_Laser_Follower_Project/Coordinate System Transformation/World Point Matrix ==
  data: WorldPoints output
function WorldPoints = StoreWorldPoints
% Update the square size to 29
squareSize = 29;

WorldPoints = [ ...
    0, 0;
    0, -squareSize;
    0, -2*squareSize;
    0, -3*squareSize;
    0, -4*squareSize;
    0, -5*squareSize;
    squareSize, 0;
    squareSize, -squareSize;
    squareSize, -2*squareSize;
    squareSize, -3*squareSize;
    squareSize, -4*squareSize;
    squareSize, -5*squareSize;
    2*squareSize, 0;
    2*squareSize, -squareSize;
    2*squareSize, -2*squareSize;
    2*squareSize, -3*squareSize;
    2*squareSize, -4*squareSize;
    2*squareSize, -5*squareSize;
    3*squareSize, 0;
    3*squareSize, -squareSize;
    3*squareSize, -2*squareSize;
    3*squareSize, -3*squareSize;
    3*squareSize, -4*squareSize;
    3*squareSize, -5*squareSize;
    4*squareSize, 0;
    4*squareSize, -squareSize;
    4*squareSize, -2*squareSize;
    4*squareSize, -3*squareSize;
    4*squareSize, -4*squareSize;
    4*squareSize, -5*squareSize;
    5*squareSize, 0;
    5*squareSize, -squareSize;
    5*squareSize, -2*squareSize;
    5*squareSize, -3*squareSize;
    5*squareSize, -4*squareSize;
    5*squareSize, -5*squareSize;
    6*squareSize, 0;
    6*squareSize, -squareSize;
    6*squareSize, -2*squareSize;
    6*squareSize, -3*squareSize;
    6*squareSize, -4*squareSize;
    6*squareSize, -5*squareSize;
    7*squareSize, 0;
    7*squareSize, -squareSize;
    7*squareSize, -2*squareSize;
    7*squareSize, -3*squareSize;
    7*squareSize, -4*squareSize;
    7*squareSize, -5*squareSize ];
end

== matlab function Automatic_Laser_Follower_Project/Coordinate System Transformation/Normalize World and Image Points ==
  data: normMatrixworld output; world input; pixel input; normMatrixImage output; ImagePointsnorm output size=[48;2]; WorldPointsnorm output size=[48;2]
function [normMatrixworld, normMatrixImage, ImagePointsnorm, WorldPointsnorm] = NormalizePoints(world, pixel)

[WorldPointsnorm,normMatrixworld] = images.geotrans.internal.normalizeControlPoints(world);

[ImagePointsnorm,normMatrixImage] = images.geotrans.internal.normalizeControlPoints(pixel);

end

== matlab function Automatic_Laser_Follower_Project/Coordinate System Transformation/2D Projective Transform ==
  data: normMatrix1 input; normMatrix2 input; xy input; uv input; tform output size=[3;3]; X output size=[96;8]; Tvec output size=[9;9]; Tinv output size=[3;3]
function [tform, X, Tvec, Tinv]  = ComputeProjectiveTransform(normMatrix1, normMatrix2, xy, uv)
    minRequiredNonCollinearPairs = 4;
    if size(uv, 1) < minRequiredNonCollinearPairs || size(xy, 1) < minRequiredNonCollinearPairs
        error('At least 4 non-collinear points are required in both input sets.');
    end
    
    % Prepare matrices for the linear system
    M = size(xy, 1);
    x = xy(:, 1);
    y = xy(:, 2);
    vec_1 = ones(M, 1);
    vec_0 = zeros(M, 1);
    u = uv(:, 1);
    v = uv(:, 2);
    
    U = [u; v];
    
    X = [x      y      vec_1  vec_0  vec_0  vec_0  -u.*x  -u.*y;
         vec_0  vec_0  vec_0  x      y      vec_1  -v.*x  -v.*y];
     
    % Solve the linear system X * Tvec = U for Tvec
    Tvec = X \ U;
    Tvec = [Tvec; 1];
    % Reshape Tvec to a 3x3 matrix, and adjust for normalization
    Tinv = reshape(Tvec, 3, 3);
    Tinv = normMatrix2 \ (Tinv * normMatrix1); % Adjust T with normalization matrices
    T = inv(Tinv);
    T = T ./ T(3, 3);
    tform = T';
end
